simulink model "a"  (R2023b)
settings: Solver=VariableStepAuto  StartTime=0.0  StopTime=10.0  RelTol=1e-3
settings Model: Creator=Administrator  LastModifiedBy=s.sh
settings SolverCC: AlgebraicLoopSolver=TrustRegion
settings DataIOCC: ReturnWorkspaceOutputs=off
settings DebuggingCC: UnconnectedInputMsg=warning  UnconnectedOutputMsg=warning  UnconnectedLineMsg=warning  ArithmeticOperatorsInVariantConditions=warning
settings ModelReferenceCC: EnableRefExpFcnMdlSchedulingChecks=on
settings SFSimCC: SimUseLocalCustomCode=off  CustomCodeUndefinedFunction=UseInterfaceOnly
settings RTWCC: RTWUseLocalCustomCode=off

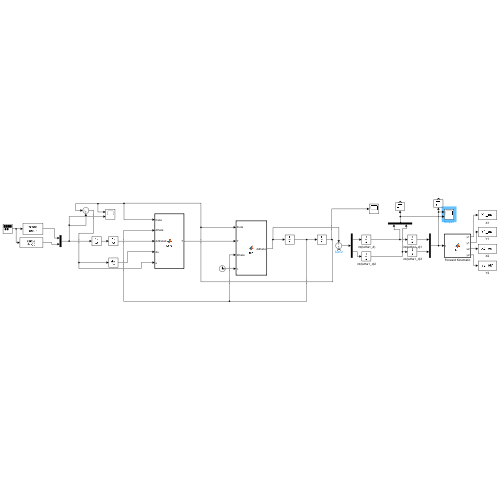
[thumbnail: Simulink's stored preview of the top-level diagram]
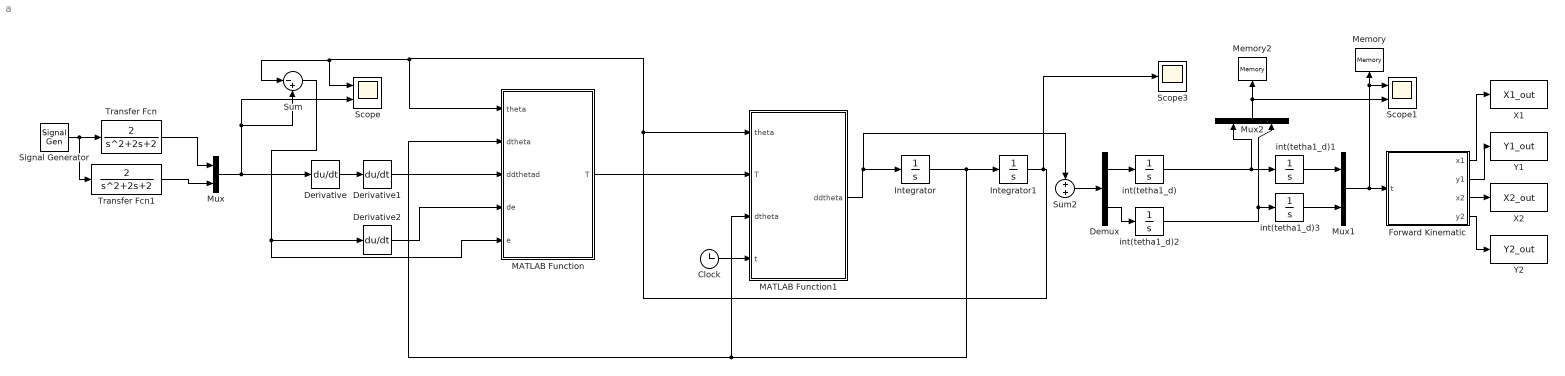
== system a ==
   int(tetha1_d){,1..3} (4 alike) : Integrator
  Clock : Clock
  Demux : Demux  Outputs=2
  Derivative : Derivative
  Derivative1 : Derivative
  Derivative2 : Derivative
  Forward Kinematic : MATLAB Function  TreatAsAtomicUnit=on
  Integrator : Integrator
  Integrator1 : Integrator
  MATLAB Function : MATLAB Function  TreatAsAtomicUnit=on
  MATLAB Function1 : MATLAB Function  TreatAsAtomicUnit=on
  Memory : Memory  InitialCondition=[0 0]
  Memory2 : Memory  InitialCondition=[0 0]
  Mux : Mux  Inputs=2
  Mux1 : Mux  Inputs=2
  Mux2 : Mux  Inputs=2
  Scope : Scope  NumInputPorts=2
  Scope1 : Scope  NumInputPorts=2
  Scope3 : Scope
  Signal Generator : SignalGenerator  Amplitude=4  Frequency=pi  Units=rad/sec
  Sum : Sum  Inputs=|-+
  Sum2 : Sum  Inputs=+|+
  Transfer Fcn : TransferFcn  Numerator=[2]  Denominator=[1 2 2]
  Transfer Fcn1 : TransferFcn  Numerator=[2]  Denominator=[1 2 2]
  X1 : ToWorkspace  VariableName=X1_out  SaveFormat=Structure With Time  SampleTime=-1
  X2 : ToWorkspace  VariableName=X2_out  SaveFormat=Structure With Time  SampleTime=-1
  Y1 : ToWorkspace  VariableName=Y1_out  SaveFormat=Structure With Time  SampleTime=-1
  Y2 : ToWorkspace  VariableName=Y2_out  SaveFormat=Structure With Time  SampleTime=-1
  wires:
  Signal Generator/1 -> Transfer Fcn1/1, Transfer Fcn/1
  Transfer Fcn/1 -> Mux/1
  Transfer Fcn1/1 -> Mux/2
  Mux/1 -> Scope/2, Sum/2, Derivative/1
  Derivative/1 -> Derivative1/1
  Derivative1/1 -> MATLAB Function/3(ddthetad)
  Derivative2/1 -> MATLAB Function/4(de)
  Sum/1 -> MATLAB Function/5(e), Derivative2/1
  MATLAB Function/1(T) -> MATLAB Function1/2(T)
  MATLAB Function1/1(ddtheta) -> Sum2/1, Integrator/1
  Integrator/1 -> MATLAB Function1/3(dtheta), MATLAB Function/2(dtheta), Integrator1/1
  Integrator1/1 -> Scope3/1, Sum/1, Scope/1, MATLAB Function/1(theta), MATLAB Function1/1(theta)
  Clock/1 -> MATLAB Function1/4(t)
  " int(tetha1_d)"/1 -> Mux2/1, " int(tetha1_d)1"/1
  Demux/1 -> " int(tetha1_d)"/1
  " int(tetha1_d)3"/1 -> Mux1/2
  Mux1/1 -> Scope1/1, Memory/1, Forward Kinematic/1(t)
  " int(tetha1_d)1"/1 -> Mux1/1
  " int(tetha1_d)2"/1 -> Mux2/2, " int(tetha1_d)3"/1
  Forward Kinematic/4(y2) -> Y2/1
  Forward Kinematic/1(x1) -> X1/1
  Forward Kinematic/3(x2) -> X2/1
  Forward Kinematic/2(y1) -> Y1/1
  Demux/2 -> " int(tetha1_d)2"/1
  Mux2/1 -> Scope1/2, Memory2/1
  Sum2/1 -> Demux/1

== matlab function a/MATLAB Function1 ==
  data: theta input; ddtheta output; T input; dtheta input; t input
function ddtheta = fcn(theta ,T , dtheta ,t)

ddtheta = [0;0];
d = 10 * sin(pi*t);
m1 = 1; m2 = 2;
L1 = 1; L2 = 1.2;
Lc1 = 0.5; Lc2 = 0.6;
I1 = 0.15; I2 = 0.3;
g = 9.8;

theta1 = theta(1); theta2 = theta(2);
dtheta1 = dtheta(1); dtheta2 = dtheta(2);


H11 = m1 * Lc1 ^2 + m2 * (Lc2^2 + L1^2 + 2 * L1 * Lc2 * cos(theta2) + I1 + I2 );
H12 = m2 * (Lc2 ^ 2 + m2 * L1 * Lc2 * cos(theta2) + I2);
H21 = H12;
H22 = m2 * Lc2 ^ 2 + I2;

c11 = -m2 * L1 * Lc2 * sin(theta2) * dtheta1;
c12 = -m2 * L1 * Lc2 * sin(theta2) * (dtheta1 + dtheta2);
c21 = m2 * L1 * Lc2 * sin (theta2) * dtheta1;

G1 = m1 * g * Lc1 * cos(theta1) + m2 * g * (L1 * cos(theta1) + Lc2* cos (theta1));
G2 = m2 * g * L2 * cos(theta1 + theta2);

H=[H11, H12;...
   H21, H22 ];
C=[c11 c12;...
    c21 0];
G=[G1; G2];

ddtheta = H\ ( T - C * dtheta - G) + d;

== matlab function a/MATLAB Function ==
  data: theta input; dtheta input; T output; ddthetad input; de input; e input
function T = smc(theta , dtheta , ddthetad , de , e)

m1 = 1; m2 = 2;
L1 = 1; L2 = 1.2;
Lc1 = 0.5; Lc2 = 0.6;
I1 = 0.15; I2 = 0.3;
g = 9.8;
D=10;

T = [0; 0];

eps = 10 * eye(2);
c = 10 * eye(2);

theta1 = theta(1); theta2 = theta(2);
dtheta1 = dtheta(1); dtheta2 = dtheta(2);


H11 = m1 * Lc1 ^2 + m2 * (Lc2^2 + L1^2 + 2 * L1 * Lc2 * cos(theta2) + I1 + I2 );
H12 = m2 * (Lc2 ^ 2 + m2 * L1 * Lc2 * cos(theta2) + I2);
H21 = H12;
H22 = m2 * Lc2 ^ 2 + I2;

c11 = -m2 * L1 * Lc2 * sin(theta2) * dtheta1;
c12 = -m2 * L1 * Lc2 * sin(theta2) * (dtheta1 + dtheta2);
c21 = m2 * L1 * Lc2 * sin (theta2) * dtheta1;

G1 = m1 * g * Lc1 * cos(theta1) + m2 * g * (L1 * cos(theta1) + Lc2* cos (theta1));
G2 = m2 * g * L2 * cos(theta1 + theta2);

H=[H11, H12;...
   H21, H22 ];
C=[c11 c12;...
    c21 0];
G=[G1; G2];

s = de + c*e;

T = H * (ddthetad + c * de + (eps + D) * sign(s) ) + C * dtheta + G;

== matlab function a/Forward Kinematic ==
  data: t input; x1 output; y1 output; x2 output; y2 output

function [x1,y1,x2,y2] = fcn(t)
m1 = 1;
m2 = 1;
l1 = 1;
lc1 = 0.5;
l2 = 1;
lc2 = 0.5;
g = 9.81;
% Joint 2 location
x1 = l1*cos(t(1));
y1 = l1*sin(t(1));
% Joint 3 location
x2 = l1*cos(t(1))+l2*cos(t(1)+t(2));
y2 = l1*sin(t(1))+l2*sin(t(1)+t(2));
